simulink model "controlador"  (R2021a)
settings: Solver=VariableStepAuto  StartTime=0.0  StopTime=Inf  RelTol=1e-3
libraries: instrumentseriallib x3
settings Model: Creator=Claudio  LastModifiedBy=mathe

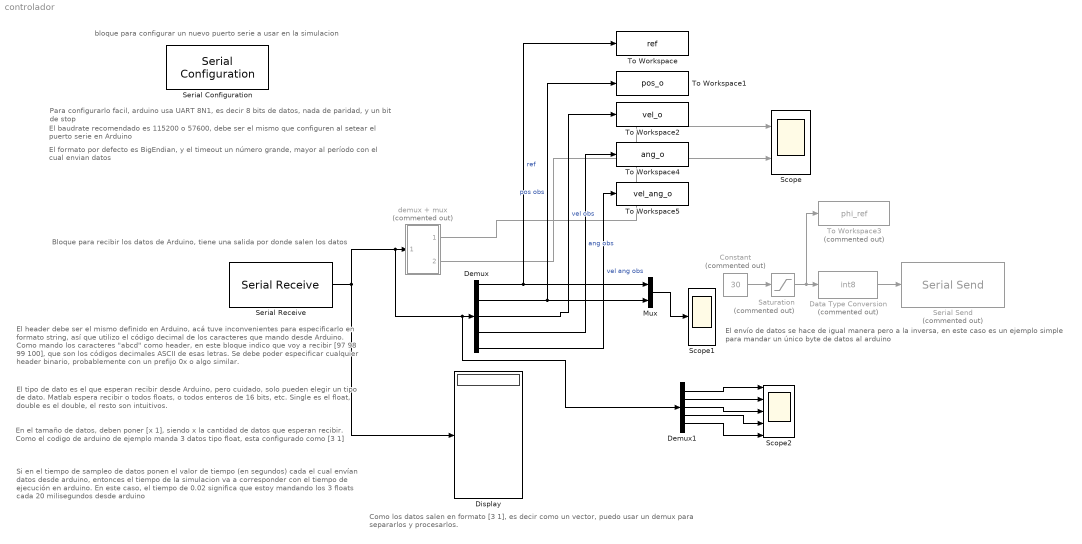
== system controlador ==
  note: El envío de datos se hace de igual manera pero a la inversa, en este caso es un ejemplo simple para mandar un único byte de datos al arduino
  note: Como los datos salen en formato [3 1], es decir como un vector, puedo usar un demux para separarlos y procesarlos.
  note: Si en el tiempo de sampleo de datos ponen el valor de tiempo (en segundos) cada el cual envían datos desde arduino, entonces el tiempo de la simulacion va a corresponder con el tiempo de ejecución en arduino. En este caso, el tiempo de 0.02 significa que estoy mandando los 3 floats cada 20 milisegundos desde arduino
  note: En el tamaño de datos, deben poner [x 1], siendo x la cantidad de datos que esperan recibir. Como el codigo de arduino de ejemplo manda 3 datos tipo float, esta configurado como [3 1]
  note: El tipo de dato es el que esperan recibir desde Arduino, pero cuidado, solo pueden elegir un tipo de dato. Matlab espera recibir o todos floats, o todos enteros de 16 bits, etc. Single es el float, double es el double, el resto son intuitivos.
  note: El header debe ser el mismo definido en Arduino, acá tuve inconvenientes para especificarlo en formato string, así que utilizo el código decimal de los caracteres que mando desde Arduino. Como mando los caracteres "abcd" como header, en este bloque indico que voy a recibir [97 98 99 100], que son los códigos decimales ASCII de esas letras. Se debe poder especificar cualquier header binario, probablemente con un prefijo 0x o algo similar.
  note: Bloque para recibir los datos de Arduino, tiene una salida por donde salen los datos
  note: El formato por defecto es BigEndian, y el timeout un número grande, mayor al período con el cual envian datos
  note: El baudrate recomendado es 115200 o 57600, debe ser el mismo que configuren al setear el puerto serie en Arduino
  note: Para configurarlo facil, arduino usa UART 8N1, es decir 8 bits de datos, nada de paridad, y un bit de stop
  note: bloque para configurar un nuevo puerto serie a usar en la simulacion
  Constant : Constant  Commented=on  Value=30
  Data Type Conversion : DataTypeConversion  Commented=on  OutDataTypeStr=int8
  Demux : Demux  Outputs=5
  Demux1 : Demux  Outputs=5
  Display : Display
  Mux : Mux  Inputs=2
  Saturation : Saturate  Commented=on  UpperLimit=45  LowerLimit=-45
  Scope : Scope  NumInputPorts=2
  Scope1 : Scope
  Scope2 : Scope  NumInputPorts=5
  Serial Configuration : instrumentseriallib/Serial Configuration  Priority=-200000  Port=COM4  ComPort=COM4  BaudRate=115200  DataBits=8  Parity=none  StopBits=1  ByteOrder=big-endian  FlowControl=none  Timeout=10  SimulateUsing=Interpreted execution  BlockInModel=on
  Serial Receive : instrumentseriallib/Serial Receive  Priority=1  Port=COM4  ComPort=COM4  DataType=single  SaveDataType=uint8  ToggleHeader=on  Header="[ 97   98   99  100 ]"  ToggleTerminator=off  Terminator=<none>  CustomTerminator=[]  ToggleDataSize=on  DataSize=[5 1]  EnableBlockingMode=on  ActionDataUnavailable=Output last received value  ActionWhenDataUnavailable=Output last received value  CustomValue=0  SampleTime=0.02  SimulateUsing=Interpreted execution  BlockInModel=on
  Serial Send : instrumentseriallib/Serial Send  Priority=1  Commented=on  Port=<Select a port...>  ComPort=<Select a port...>  Header=[]  Terminator=<none>  CustomTerminator=[]  EnableBlockingMode=on  SimulateUsing=Interpreted execution  BlockInModel=on
  To Workspace : ToWorkspace  VariableName=ref  SampleTime=-1
      settings: Save2DSignal=2-D array (concatenate along first dimension)
  To Workspace1 : ToWorkspace  VariableName=pos_o  SampleTime=-1
      settings: Save2DSignal=2-D array (concatenate along first dimension)
  To Workspace2 : ToWorkspace  VariableName=vel_o  SampleTime=-1
      settings: Save2DSignal=2-D array (concatenate along first dimension)
  To Workspace3 : ToWorkspace  Commented=on  VariableName=phi_ref  SampleTime=0.02
      settings: Save2DSignal=2-D array (concatenate along first dimension)
  To Workspace4 : ToWorkspace  VariableName=ang_o  SampleTime=-1
      settings: Save2DSignal=2-D array (concatenate along first dimension)
  To Workspace5 : ToWorkspace  VariableName=vel_ang_o  SampleTime=-1
      settings: Save2DSignal=2-D array (concatenate along first dimension)
  demux + mux : Subsystem  Commented=on
  wires:
  Serial Receive/1 -> Display/1, Demux1/1, Demux/1, demux + mux/1(In1)
  Data Type Conversion/1 -> Serial Send/1
  Constant/1 -> Saturation/1
  Saturation/1 -> To Workspace3/1, Data Type Conversion/1
  demux + mux/1(Out1) -> Scope/1
  demux + mux/2(Out2) -> Scope/2
  Demux/1 -> To Workspace/1, Mux/1  "ref"
  Demux/3 -> To Workspace2/1  "vel obs"
  Demux/2 -> To Workspace1/1, Mux/2  "pos obs"
  Demux/4 -> To Workspace4/1  "ang obs"
  Demux1/2 -> Scope2/2
  Demux1/5 -> Scope2/5
  Demux1/4 -> Scope2/4
  Demux1/3 -> Scope2/3
  Demux1/1 -> Scope2/1
  Demux/5 -> To Workspace5/1  "vel ang obs"
  Mux/1 -> Scope1/1

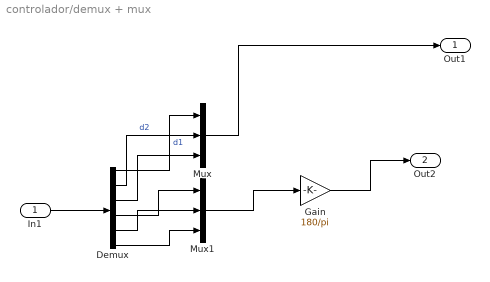
== system controlador/demux + mux ==
  In1 : Inport
  Demux : Demux  Outputs=6
  Gain : Gain  Gain=180/pi
  Mux : Mux  Inputs=3
  Mux1 : Mux  Inputs=3
  Out1 : Outport
  Out2 : Outport  Port=2
  wires:
  Demux/2 -> Mux/2  "d2"
  Demux/3 -> Mux/3
  Demux/1 -> Mux/1  "d1"
  Demux/6 -> Mux1/3
  Demux/5 -> Mux1/2
  Demux/4 -> Mux1/1
  In1/1 -> Demux/1
  Mux/1 -> Out1/1
  Mux1/1 -> Gain/1
  Gain/1 -> Out2/1
